simulink model "FSPContinuousSimulink"  (R2023b)
settings: Solver=VariableStepAuto  StartTime=0.0  StopTime=40  RelTol=1e-3
values from neighbouring files (symbols this model uses):
  denp = [3 1]    [FSPContinuous.m]
  h = 6.5    [FSPContinuous.m]
  nump = 2    [FSPContinuous.m]
libraries: cstblocks x5
settings Model: Creator=klysm  LastModifiedBy=klysm

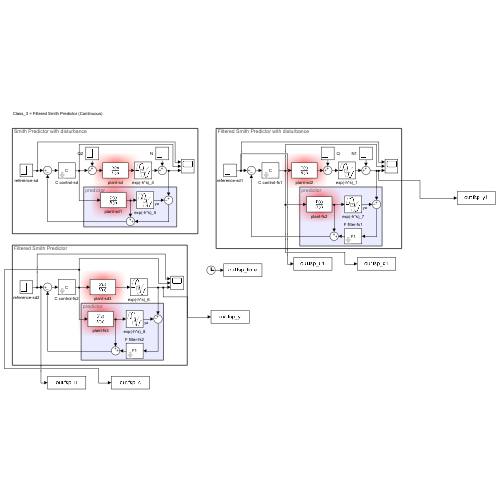
[thumbnail: Simulink's stored preview of the top-level diagram]
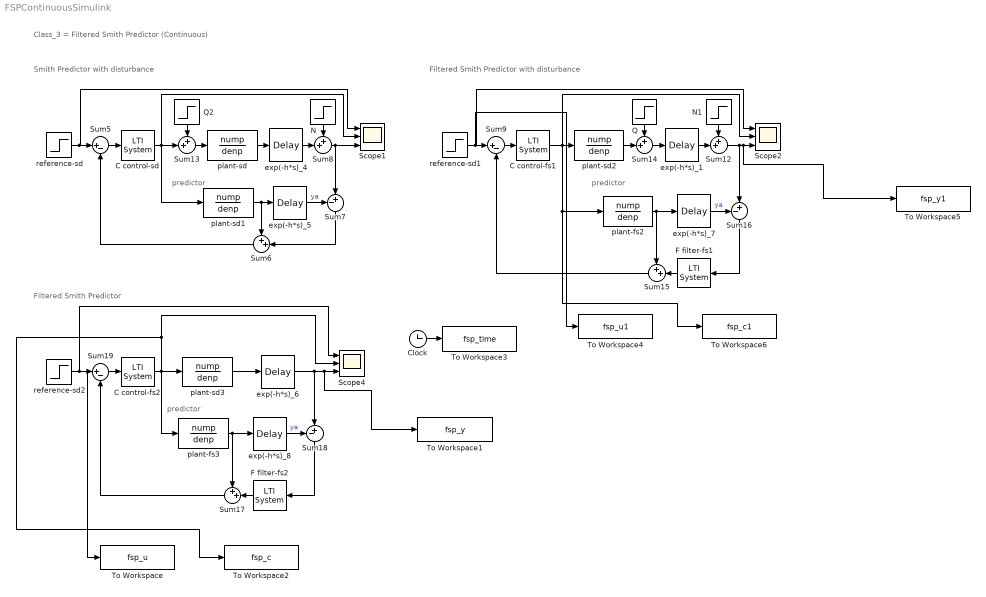
== system FSPContinuousSimulink ==
  note: Class_3 = Filtered Smith Predictor (Continuous)
  note: predictor
  note: Smith Predictor with disturbance
  note: Filtered Smith Predictor with disturbance
  note: Filtered Smith Predictor
  note: predictor
  note: predictor
  C control-fs1 : cstblocks/LTI System  sys=C  IC=[]  PadeOrder=0
  C control-fs2 : cstblocks/LTI System  sys=C  IC=[]  PadeOrder=0
  C control-sd : cstblocks/LTI System  sys=C  IC=[]  PadeOrder=0
  Clock : Clock
  F filter-fs1 : cstblocks/LTI System  sys=F1  IC=[]  PadeOrder=0
  F filter-fs2 : cstblocks/LTI System  sys=F1  IC=[]  PadeOrder=0
  N : Step  Time=20  After=0.2  SampleTime=0
  N1 : Step  Time=20  After=0.2  SampleTime=0
  Q : Step  Time=10  After=0.2  SampleTime=0
  Q2 : Step  Time=10  After=0.2  SampleTime=0
  Scope1 : Scope  NumInputPorts=3
  Scope2 : Scope  NumInputPorts=3
  Scope4 : Scope  NumInputPorts=3
  Sum{6,8,12..15,17} (7 alike) : Sum  Inputs=++|
  Sum16 : Sum  Inputs=-+|
  Sum18 : Sum  Inputs=-+|
  Sum19 : Sum  Inputs=|+-
  Sum5 : Sum  Inputs=|+-
  Sum7 : Sum  Inputs=-+|
  Sum9 : Sum  Inputs=|+-
  To Workspace : ToWorkspace  VariableName=fsp_u  SampleTime=-1
  To Workspace1 : ToWorkspace  VariableName=fsp_y  SampleTime=-1
  To Workspace2 : ToWorkspace  VariableName=fsp_c  SampleTime=-1
  To Workspace3 : ToWorkspace  VariableName=fsp_time  SampleTime=-1
  To Workspace4 : ToWorkspace  VariableName=fsp_u1  SampleTime=-1
  To Workspace5 : ToWorkspace  VariableName=fsp_y1  SampleTime=-1
  To Workspace6 : ToWorkspace  VariableName=fsp_c1  SampleTime=-1
  exp(-h*s)_{1,4..8} (6 alike) : TransportDelay  DelayTime=h
  plant-fs2 : TransferFcn  Numerator=nump  Denominator=denp
  plant-fs3 : TransferFcn  Numerator=nump  Denominator=denp
  plant-sd{,1..3} (4 alike) : TransferFcn  Numerator=nump  Denominator=denp
  reference-sd : Step  Time=0  SampleTime=0
  reference-sd1 : Step  Time=0  SampleTime=0
  reference-sd2 : Step  Time=0  SampleTime=0
  wires:
  Q2/1 -> Sum13/1
  Sum13/1 -> plant-sd/1
  Sum5/1 -> C control-sd/1
  N/1 -> Sum8/1
  Sum8/1 -> Scope1/3, Sum7/2
  exp(-h*s)_5/1 -> Sum7/1  "ya"
  plant-sd1/1 -> Sum6/1, exp(-h*s)_5/1
  Sum6/1 -> Sum5/2
  Sum7/1 -> Sum6/2
  reference-sd/1 -> Scope1/1, Sum5/1
  exp(-h*s)_4/1 -> Sum8/2
  plant-sd/1 -> exp(-h*s)_4/1
  C control-sd/1 -> Sum13/2, Scope1/2, plant-sd1/1
  C control-fs1/1 -> plant-sd2/1, To Workspace6/1, plant-fs2/1, Scope2/2
  Sum9/1 -> C control-fs1/1
  N1/1 -> Sum12/1
  reference-sd1/1 -> To Workspace4/1, Scope2/1, Sum9/1
  exp(-h*s)_1/1 -> Sum12/2
  Sum15/1 -> Sum9/2
  Sum12/1 -> To Workspace5/1, Scope2/3, Sum16/2
  F filter-fs1/1 -> Sum15/2
  plant-fs2/1 -> exp(-h*s)_7/1, Sum15/1
  exp(-h*s)_7/1 -> Sum16/1  "ya"
  Sum16/1 -> F filter-fs1/1
  Sum18/1 -> F filter-fs2/1
  F filter-fs2/1 -> Sum17/2
  plant-sd3/1 -> exp(-h*s)_6/1
  reference-sd2/1 -> To Workspace/1, Scope4/1, Sum19/1
  plant-fs3/1 -> exp(-h*s)_8/1, Sum17/1
  exp(-h*s)_6/1 -> To Workspace1/1, Scope4/3, Sum18/2
  Sum19/1 -> C control-fs2/1
  Sum17/1 -> Sum19/2
  C control-fs2/1 -> plant-sd3/1, To Workspace2/1, Scope4/2, plant-fs3/1
  exp(-h*s)_8/1 -> Sum18/1  "ya"
  Clock/1 -> To Workspace3/1
  Q/1 -> Sum14/1
  plant-sd2/1 -> Sum14/2
  Sum14/1 -> exp(-h*s)_1/1
